simulink model "SuspensionSystem"  (R2020a)
settings: Solver=VariableStepAuto  StartTime=0.0  StopTime=100.0  RelTol=1e-3
PostLoadFcn:
  | m1=2500;
  | m2=320;
  | k1=80000;
  | k2=500000;
  | b=320;
settings Model: DataDictionary=DDict.sldd  Creator=Hp  LastModifiedBy=Hp
settings DataIOCC: ExternalInput=[t,signal]  LoadExternalInput=on

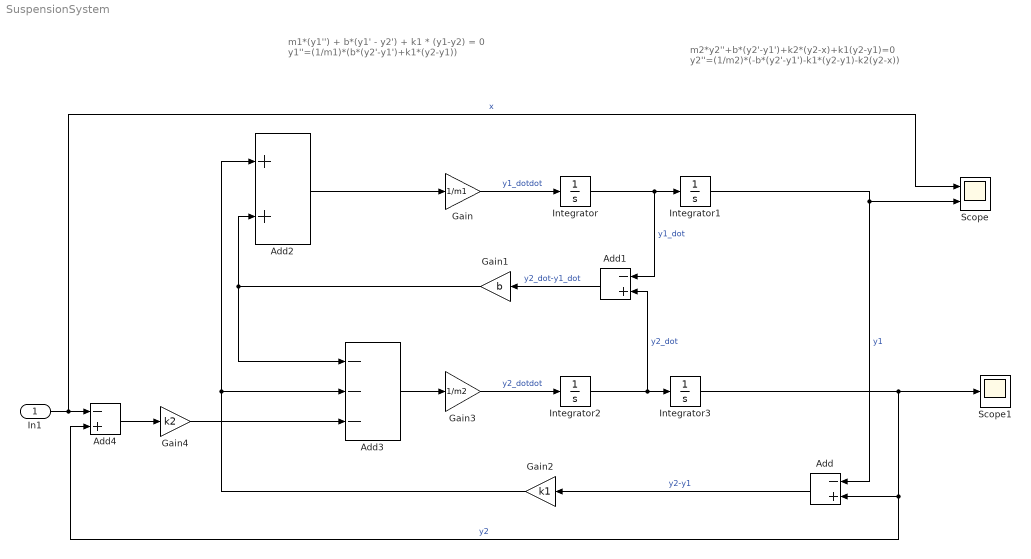
== system SuspensionSystem ==
  note: m2*y2''+b*(y2'-y1')+k2*(y2-x)+k1(y2-y1)=0
      |
      | y2''=(1/m2)*(-b*(y2'-y1')-k1*(y2-y1)-k2(y2-x))
  note: m1*(y1'') + b*(y1' - y2') + k1 * (y1-y2) = 0
      |
      | y1''=(1/m1)*(b*(y2'-y1')+k1*(y2-y1))
  In1 : Inport
  Add : Sum  Inputs=-+
  Add1 : Sum  Inputs=-+
  Add2 : Sum
  Add3 : Sum  Inputs=---
  Add4 : Sum  Inputs=-+
  Gain : Gain  Gain=1/m1
  Gain1 : Gain  Gain=b
  Gain2 : Gain  Gain=k1
  Gain3 : Gain  Gain=1/m2
  Gain4 : Gain  Gain=k2
  Integrator{,1..3} (4 alike) : Integrator
  Scope : Scope  NumInputPorts=2
  Scope1 : Scope
  wires:
  Integrator/1 -> Add1/1, Integrator1/1  "y1_dot"
  Gain/1 -> Integrator/1  "y1_dotdot"
  Integrator1/1 -> Scope/2, Add/1  "y1"
  Gain3/1 -> Integrator2/1  "y2_dotdot"
  Integrator2/1 -> Add1/2, Integrator3/1  "y2_dot"
  Integrator3/1 -> Scope1/1, Add4/2, Add/2  "y2"
  Add/1 -> Gain2/1  "y2-y1"
  Add1/1 -> Gain1/1  "y2_dot-y1_dot"
  Add2/1 -> Gain/1
  Gain1/1 -> Add2/2, Add3/1
  Gain2/1 -> Add2/1, Add3/2
  Add3/1 -> Gain3/1
  In1/1 -> Scope/1, Add4/1  "x"
  Add4/1 -> Gain4/1
  Gain4/1 -> Add3/3
